simulink model "FullSystemCyclesv2"  (R2025b)
settings: Solver=VariableStepAuto  StartTime=0.0  StopTime=60*60  RelTol=1e-3
libraries: fl_lib x65, nesl_utility x42, SimscapeFluids_lib x13, simulink x1
(part 2 of 2)

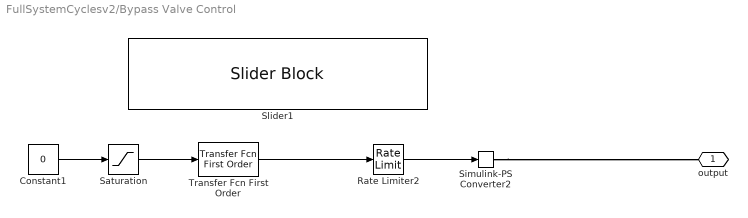
== system FullSystemCyclesv2/Bypass Valve Control ==
  Constant1 : Constant  Value=0  OutMin=0  OutMax=1  OutDataTypeStr=double
  Rate Limiter2 : RateLimiter  RisingSlewLimit=0.02  FallingSlewLimit=-0.02  SampleTimeMode=inherited
  Saturation : Saturate
  Simulink-PS Converter2 : nesl_utility/Simulink-PS Converter  PhysicalDomain=network_engine_domain  SubClassName=ps_input  LeftPortType=input  RightPortType=output  PseudoPeriodic=off  Frequencies=[]  NoiseDistribution=none  NoiseParameters=[]  Unit=1  AffineConversion=off  FilteringAndDerivatives=provide  SimscapeFilterOrder=1  InputFilterTimeConstant=0.001  UdotUserProvided=0
  Slider1 : SliderBlock  ScaleMax=1  TickInterval=0.1
  Transfer Fcn First Order : simulink/Discrete/Transfer Fcn First Order  PoleZ=0.9802  ICPrevOutput=0.0  DoSatur=off
  output : PMIOPort  Side=Right
  wires:
  Constant1/1 -> Saturation/1
  Saturation/1 -> Transfer Fcn First Order/1
  Transfer Fcn First Order/1 -> Rate Limiter2/1
  Rate Limiter2/1 -> Simulink-PS Converter2/1
  connections:
  Simulink-PS Converter2/RConn1 -- output/RConn1
